simulink library "telemetrySubsystem"  (R2021b)
settings: Solver=VariableStepAuto  StartTime=0.0  StopTime=10.0  RelTol=1e-3
libraries: aerolibutil x4, conversionsLib x2
settings Model: Creator=mat  LastModifiedBy=mat

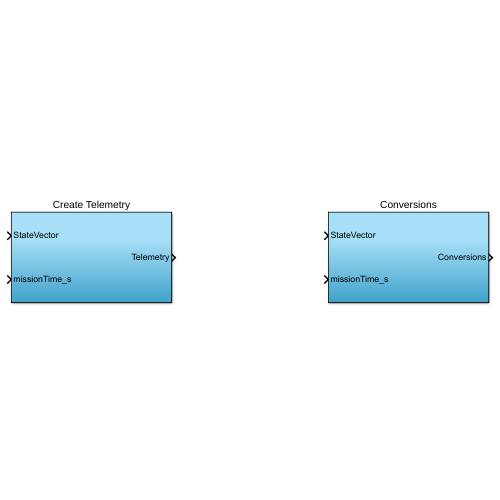
[thumbnail: Simulink's stored preview of the top-level diagram]
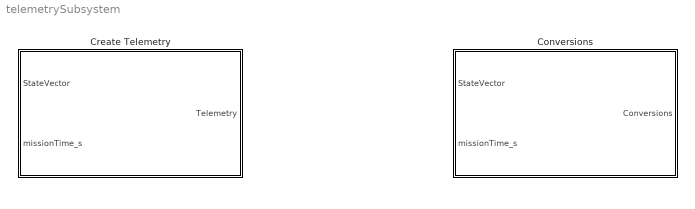
== system telemetrySubsystem ==
  Conversions : Subsystem
  Create Telemetry : Subsystem

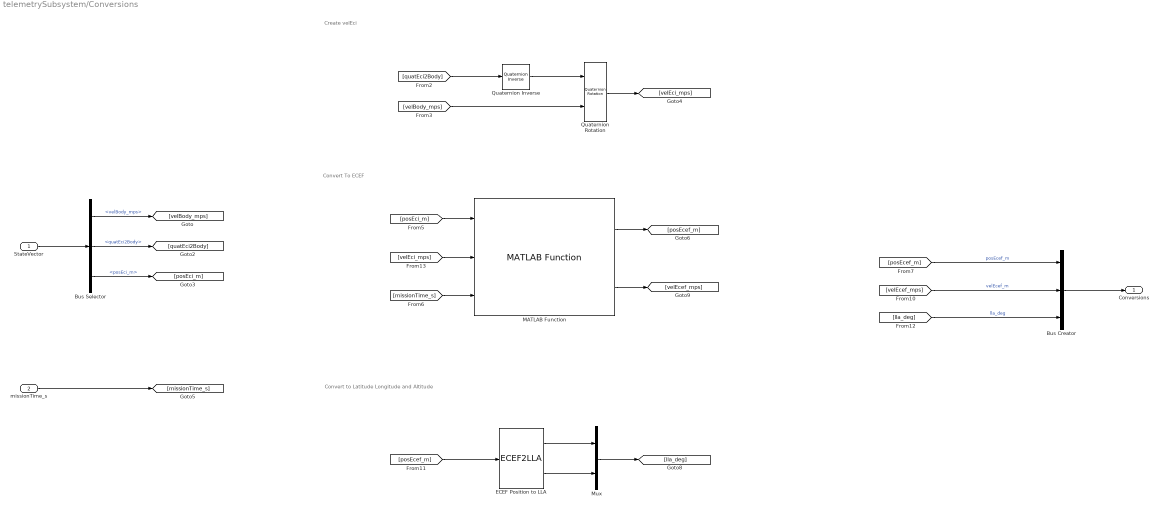
== system telemetrySubsystem/Conversions ==
  note: Create velEci
  note: Convert To ECEF
  note: Convert to Latitude Longitude and Altitude
  StateVector : Inport  OutDataTypeStr=Bus: StateVector_BusType
  missionTime_s : Inport  Port=2
  Bus Creator : BusCreator  Inputs=3  OutDataTypeStr=Bus: Conversions_BusType  NonVirtualBus=on
      settings: InheritFromInputs=off
  Bus Selector : BusSelector  OutputSignals=velBody_mps,quatEci2Body,posEci_m
  ECEF Position to LLA : ECEF2LLA
  MATLAB Function : conversionsLib/MATLAB Function  SystemSampleTime=-1  VariantActivationTime=update diagram  Latency=0  AutoFrameSizeCalculation=off
  Mux : Mux  Inputs=2
  Quaternion Inverse : aerolibutil/Quaternion Inverse
  Quaternion Rotation : aerolibutil/Quaternion Rotation
  Conversions : Outport  OutDataTypeStr=Bus: Conversions_BusType
  wires:
  Bus Creator/1 -> Conversions/1
  [lla_deg] -> Bus Creator/3  "lla_deg"
  [velEcef_mps] -> Bus Creator/2  "velEcef_m"
  [posEcef_m] -> Bus Creator/1  "posEcef_m"
  Mux/1 -> [lla_deg]
  ECEF Position to LLA/2 -> Mux/2
  ECEF Position to LLA/1 -> Mux/1
  [posEcef_m] -> ECEF Position to LLA/1
  MATLAB Function/1 -> [posEcef_m]
  [missionTime_s] -> MATLAB Function/3
  missionTime_s/1 -> [missionTime_s]
  [posEci_m] -> MATLAB Function/1
  Quaternion Rotation/1 -> [velEci_mps]
  [velBody_mps] -> Quaternion Rotation/2
  Quaternion Inverse/1 -> Quaternion Rotation/1
  [quatEci2Body] -> Quaternion Inverse/1
  Bus Selector/3 -> [posEci_m]  "<posEci_m>"
  Bus Selector/2 -> [quatEci2Body]  "<quatEci2Body>"
  Bus Selector/1 -> [velBody_mps]  "<velBody_mps>"
  StateVector/1 -> Bus Selector/1
  [velEci_mps] -> MATLAB Function/2
  MATLAB Function/2 -> [velEcef_mps]

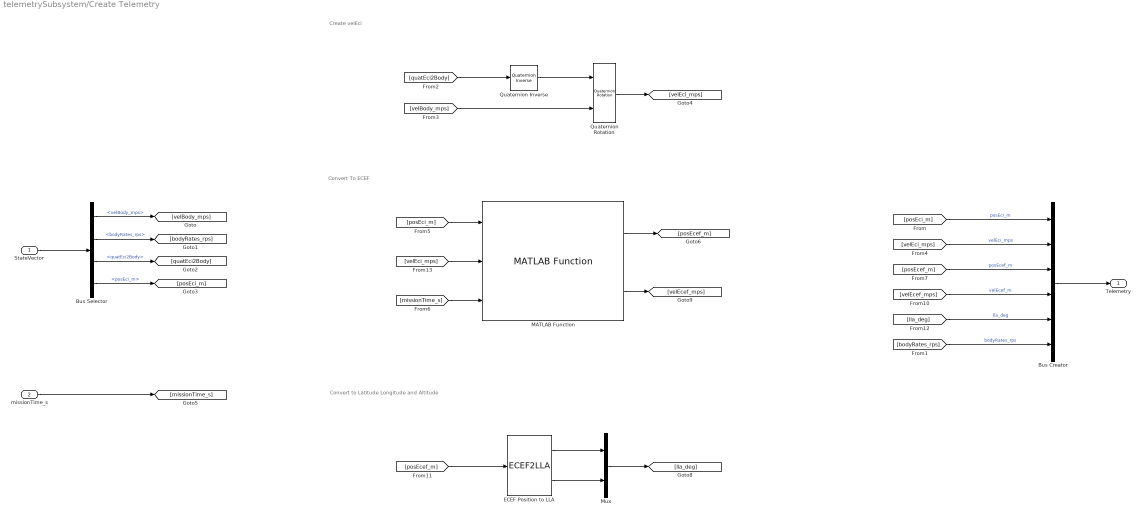
== system telemetrySubsystem/Create Telemetry ==
  note: Create velEci
  note: Convert To ECEF
  note: Convert to Latitude Longitude and Altitude
  StateVector : Inport  OutDataTypeStr=Bus: StateVector_BusType
  missionTime_s : Inport  Port=2
  Bus Creator : BusCreator  Inputs=6  OutDataTypeStr=Bus: Telemetry_BusType  NonVirtualBus=on
      settings: InheritFromInputs=off
  Bus Selector : BusSelector  OutputSignals=velBody_mps,bodyRates_rps,quatEci2Body,posEci_m
  ECEF Position to LLA : ECEF2LLA
  MATLAB Function : conversionsLib/MATLAB Function  SystemSampleTime=-1  VariantActivationTime=update diagram  Latency=0  AutoFrameSizeCalculation=off
  Mux : Mux  Inputs=2
  Quaternion Inverse : aerolibutil/Quaternion Inverse
  Quaternion Rotation : aerolibutil/Quaternion Rotation
  Telemetry : Outport  OutDataTypeStr=Bus: Telemetry_BusType
  wires:
  Mux/1 -> [lla_deg]
  ECEF Position to LLA/2 -> Mux/2
  ECEF Position to LLA/1 -> Mux/1
  [posEcef_m] -> ECEF Position to LLA/1
  MATLAB Function/1 -> [posEcef_m]
  [missionTime_s] -> MATLAB Function/3
  missionTime_s/1 -> [missionTime_s]
  [posEci_m] -> MATLAB Function/1
  Quaternion Rotation/1 -> [velEci_mps]
  [velBody_mps] -> Quaternion Rotation/2
  Quaternion Inverse/1 -> Quaternion Rotation/1
  [quatEci2Body] -> Quaternion Inverse/1
  Bus Selector/4 -> [posEci_m]  "<posEci_m>"
  Bus Selector/3 -> [quatEci2Body]  "<quatEci2Body>"
  [bodyRates_rps] -> Bus Creator/6  "bodyRates_rps"
  Bus Selector/2 -> [bodyRates_rps]  "<bodyRates_rps>"
  Bus Selector/1 -> [velBody_mps]  "<velBody_mps>"
  StateVector/1 -> Bus Selector/1
  [lla_deg] -> Bus Creator/5  "lla_deg"
  [posEci_m] -> Bus Creator/1  "posEci_m"
  [velEcef_mps] -> Bus Creator/4  "velEcef_m"
  [posEcef_m] -> Bus Creator/3  "posEcef_m"
  [velEci_mps] -> Bus Creator/2  "velEci_mps"
  Bus Creator/1 -> Telemetry/1
  [velEci_mps] -> MATLAB Function/2
  MATLAB Function/2 -> [velEcef_mps]
